simulink model "EPSArchitecture"  (R2024b)
settings: Solver=VariableStepAuto  StartTime=0.0  StopTime=10.0  RelTol=1e-3
undefined symbols (not defined in the file): I, V
settings Model: Creator=Ameya  LastModifiedBy=Ameya

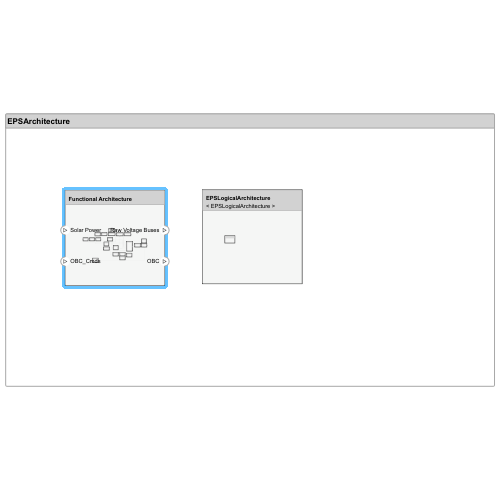
[thumbnail: Simulink's stored preview of the top-level diagram]
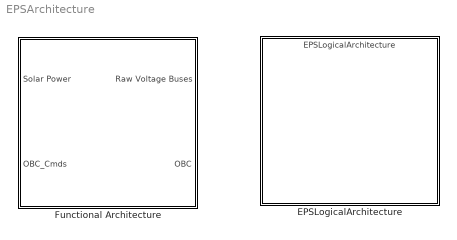
== system EPSArchitecture ==
  EPSLogicalArchitecture : ModelReference  ModelNameDialog=EPSLogicalArchitecture.slx  SimulationMode=Normal  ModelReferenceVersion=1.2
      settings: PortSchema="{\"entries\":[{\"content\":{\"headerSize\":38,\"margin\":15,\"minimumSpacing\":25,\"sides\":[{\"content\":{},\"type\":\"ConnectorPlacement.EquallySpacedRectSide\",\"uuid\":\"16a4dedc-e801-4c3c-832f-0dd2c6390a3f\"},{\"content\":{\"side\":\"RIGHT\"},\"type\":\"ConnectorPlacement.EquallySpacedRectSide\",\"uuid\":\"ee639550-12e3-4867-a673-c6f4541c780d\"},{\"content\":{\"side\":\"TOP\"},\"type\":\"ConnectorPlacement.EquallySpacedRectSide\",\"uuid\":\"10f850c7-9a2f-4ef9-b95e-dde16675c468\"}]},\"type\":\"ConnectorPlacement.EquallySpacedConnector\",\"uuid\":\"a54e4fd9-9c39-4006-b310-35c5d04543b4\"}],\"packageUris\":[\"http://schema.mathworks.com/mf0/Connector/R2020b\"],\"version\":\"1.0\"}"
  Functional Architecture : Subsystem
      settings: PortSchema="{\"entries\":[{\"content\":{\"headerSize\":26,\"margin\":15,\"minimumSpacing\":25,\"sides\":[{\"content\":{\"connectorIds\":[\"In1\",\"In2\"]},\"type\":\"ConnectorPlacement.EquallySpacedRectSide\",\"uuid\":\"94509738-6f31-4862-b12a-7ef357457276\"},{\"content\":{\"connectorIds\":[\"Out1\",\"Out2\"],\"side\":\"RIGHT\"},\"type\":\"ConnectorPlacement.EquallySpacedRectSide\",\"uuid\":\"5e6a1bf4-2d31-4a4e-ab5c-eea221f5967b\"},{\"content\":{\"side\":\"TOP\"},\"type\":\"ConnectorPlacement.EquallySpacedRectSide\",\"uuid\":\"a8cbd51e-1f9f-4875-b1c6-5db1e209e4cb\"}]},\"type\":\"ConnectorPlacement.EquallySpacedConnector\",\"uuid\":\"3c3107f4-6377-41ce-bc87-a3d6aad033f0\"}],\"packageUris\":[\"http://schema.mathworks.com/mf0/Connector/R2020b\"],\"version\":\"1.0\"}"

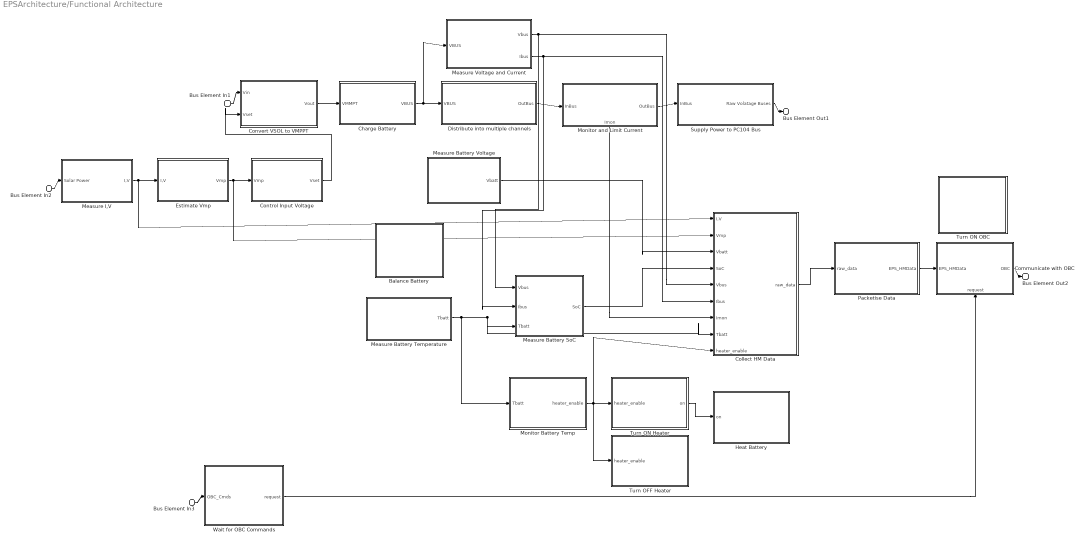
== system EPSArchitecture/Functional Architecture ==
  Bus Element In1 : Inport  PortName=Solar Power
  Bus Element In2 : Inport  PortName=Solar Power
  Bus Element In3 : Inport  Port=2  PortName=OBC_Cmds
  Balance Battery : Subsystem
      settings: PortSchema="{\"entries\":[{\"content\":{\"headerSize\":26,\"margin\":15,\"minimumSpacing\":25,\"sides\":[{\"content\":{},\"type\":\"ConnectorPlacement.EquallySpacedRectSide\",\"uuid\":\"94509738-6f31-4862-b12a-7ef357457276\"},{\"content\":{\"side\":\"RIGHT\"},\"type\":\"ConnectorPlacement.EquallySpacedRectSide\",\"uuid\":\"5e6a1bf4-2d31-4a4e-ab5c-eea221f5967b\"},{\"content\":{\"side\":\"TOP\"},\"type\":\"ConnectorPlacement.EquallySpacedRectSide\",\"uuid\":\"a8cbd51e-1f9f-4875-b1c6-5db1e209e4cb\"}]},\"type\":\"ConnectorPlacement.EquallySpacedConnector\",\"uuid\":\"3c3107f4-6377-41ce-bc87-a3d6aad033f0\"}],\"packageUris\":[\"http://schema.mathworks.com/mf0/Connector/R2020b\"],\"version\":\"1.0\"}"
  Charge Battery : Subsystem
      settings: PortSchema="{\"entries\":[{\"content\":{\"headerSize\":26,\"margin\":15,\"minimumSpacing\":25,\"sides\":[{\"content\":{\"connectorIds\":[\"In1\"]},\"type\":\"ConnectorPlacement.EquallySpacedRectSide\",\"uuid\":\"94509738-6f31-4862-b12a-7ef357457276\"},{\"content\":{\"connectorIds\":[\"Out1\"],\"side\":\"RIGHT\"},\"type\":\"ConnectorPlacement.EquallySpacedRectSide\",\"uuid\":\"5e6a1bf4-2d31-4a4e-ab5c-eea221f5967b\"},{\"content\":{\"side\":\"TOP\"},\"type\":\"ConnectorPlacement.EquallySpacedRectSide\",\"uuid\":\"a8cbd51e-1f9f-4875-b1c6-5db1e209e4cb\"}]},\"type\":\"ConnectorPlacement.EquallySpacedConnector\",\"uuid\":\"3c3107f4-6377-41ce-bc87-a3d6aad033f0\"}],\"packageUris\":[\"http://schema.mathworks.com/mf0/Connector/R2020b\"],\"version\":\"1.0\"}"
  Collect HM Data : Subsystem
      settings: PortSchema="{\"entries\":[{\"content\":{\"headerSize\":26,\"margin\":15,\"minimumSpacing\":25,\"sides\":[{\"content\":{\"connectorIds\":[\"In2\",\"In3\",\"In7\",\"In5\",\"In4\",\"In6\",\"In1\",\"In8\",\"In9\"]},\"type\":\"ConnectorPlacement.EquallySpacedRectSide\",\"uuid\":\"94509738-6f31-4862-b12a-7ef357457276\"},{\"content\":{\"connectorIds\":[\"Out1\"],\"side\":\"RIGHT\"},\"type\":\"ConnectorPlacement.EquallySpacedRectSide\",\"uuid\":\"5e6a1bf4-2d31-4a4e-ab5c-eea221f5967b\"},{\"content\":{\"side\":\"TOP\"},\"type\":\"ConnectorPlacement.EquallySpacedRectSide\",\"uuid\":\"a8cbd51e-1f9f-4875-b1c6-5db1e209e4cb\"},{\"content\":{\"side\":\"BOTTOM\"},\"type\":\"ConnectorPlacement.EquallySpacedRectSide\",\"uuid\":\"894155b8-c903-4898-a21f-10b96531ddc8\"}]},\"type\":\"ConnectorPlacement.EquallySpacedConnector\",\"uuid\":\"3c3107f4-6377-41ce-bc87-a3d6aad033f0\"}],\"packageUris\":[\"http://schema.mathworks.com/mf0/Connector/R2020b\"],\"version\":\"1.0\"}"
  Communicate with OBC : Subsystem
      settings: PortSchema="{\"entries\":[{\"content\":{\"headerSize\":26,\"margin\":15,\"minimumSpacing\":25,\"sides\":[{\"content\":{\"connectorIds\":[\"In2\"]},\"type\":\"ConnectorPlacement.EquallySpacedRectSide\",\"uuid\":\"94509738-6f31-4862-b12a-7ef357457276\"},{\"content\":{\"connectorIds\":[\"Out1\"],\"side\":\"RIGHT\"},\"type\":\"ConnectorPlacement.EquallySpacedRectSide\",\"uuid\":\"5e6a1bf4-2d31-4a4e-ab5c-eea221f5967b\"},{\"content\":{\"side\":\"TOP\"},\"type\":\"ConnectorPlacement.EquallySpacedRectSide\",\"uuid\":\"a8cbd51e-1f9f-4875-b1c6-5db1e209e4cb\"},{\"content\":{\"connectorIds\":[\"In1\"],\"side\":\"BOTTOM\"},\"type\":\"ConnectorPlacement.EquallySpacedRectSide\",\"uuid\":\"5c85cd8d-b96f-4b01-934b-f3c1b61044cb\"}]},\"type\":\"ConnectorPlacement.EquallySpacedConnector\",\"uuid\":\"3c3107f4-6377-41ce-bc87-a3d6aad033f0\"}],\"packageUris\":[\"http://schema.mathworks.com/mf0/Connector/R2020b\"],\"version\":\"1.0\"}"
  Control Input Voltage : Subsystem
      settings: PortSchema="{\"entries\":[{\"content\":{\"headerSize\":26,\"margin\":15,\"minimumSpacing\":25,\"sides\":[{\"content\":{\"connectorIds\":[\"In1\"]},\"type\":\"ConnectorPlacement.EquallySpacedRectSide\",\"uuid\":\"94509738-6f31-4862-b12a-7ef357457276\"},{\"content\":{\"connectorIds\":[\"Out1\"],\"side\":\"RIGHT\"},\"type\":\"ConnectorPlacement.EquallySpacedRectSide\",\"uuid\":\"5e6a1bf4-2d31-4a4e-ab5c-eea221f5967b\"},{\"content\":{\"side\":\"TOP\"},\"type\":\"ConnectorPlacement.EquallySpacedRectSide\",\"uuid\":\"a8cbd51e-1f9f-4875-b1c6-5db1e209e4cb\"}]},\"type\":\"ConnectorPlacement.EquallySpacedConnector\",\"uuid\":\"3c3107f4-6377-41ce-bc87-a3d6aad033f0\"}],\"packageUris\":[\"http://schema.mathworks.com/mf0/Connector/R2020b\"],\"version\":\"1.0\"}"
  Convert VSOL to VMPPT : Subsystem
      settings: PortSchema="{\"entries\":[{\"content\":{\"headerSize\":26,\"margin\":15,\"minimumSpacing\":25,\"sides\":[{\"content\":{\"connectorIds\":[\"In2\",\"In1\"]},\"type\":\"ConnectorPlacement.EquallySpacedRectSide\",\"uuid\":\"94509738-6f31-4862-b12a-7ef357457276\"},{\"content\":{\"connectorIds\":[\"Out1\"],\"side\":\"RIGHT\"},\"type\":\"ConnectorPlacement.EquallySpacedRectSide\",\"uuid\":\"5e6a1bf4-2d31-4a4e-ab5c-eea221f5967b\"},{\"content\":{\"side\":\"TOP\"},\"type\":\"ConnectorPlacement.EquallySpacedRectSide\",\"uuid\":\"a8cbd51e-1f9f-4875-b1c6-5db1e209e4cb\"},{\"content\":{\"side\":\"BOTTOM\"},\"type\":\"ConnectorPlacement.EquallySpacedRectSide\",\"uuid\":\"4bc2357f-6cbf-4a1a-8384-978abe31c3d6\"}]},\"type\":\"ConnectorPlacement.EquallySpacedConnector\",\"uuid\":\"3c3107f4-6377-41ce-bc87-a3d6aad033f0\"}],\"packageUris\":[\"http://schema.mathworks.com/mf0/Connector/R2020b\"],\"version\":\"1.0\"}"
  Distribute into multiple channels : Subsystem
      settings: PortSchema="{\"entries\":[{\"content\":{\"headerSize\":26,\"margin\":15,\"minimumSpacing\":25,\"sides\":[{\"content\":{\"connectorIds\":[\"In1\"]},\"type\":\"ConnectorPlacement.EquallySpacedRectSide\",\"uuid\":\"94509738-6f31-4862-b12a-7ef357457276\"},{\"content\":{\"connectorIds\":[\"Out1\"],\"side\":\"RIGHT\"},\"type\":\"ConnectorPlacement.EquallySpacedRectSide\",\"uuid\":\"5e6a1bf4-2d31-4a4e-ab5c-eea221f5967b\"},{\"content\":{\"side\":\"TOP\"},\"type\":\"ConnectorPlacement.EquallySpacedRectSide\",\"uuid\":\"a8cbd51e-1f9f-4875-b1c6-5db1e209e4cb\"},{\"content\":{\"side\":\"BOTTOM\"},\"type\":\"ConnectorPlacement.EquallySpacedRectSide\",\"uuid\":\"75e56ff6-a338-4e40-9de2-d2fe93eef496\"}]},\"type\":\"ConnectorPlacement.EquallySpacedConnector\",\"uuid\":\"3c3107f4-6377-41ce-bc87-a3d6aad033f0\"}],\"packageUris\":[\"http://schema.mathworks.com/mf0/Connector/R2020b\"],\"version\":\"1.0\"}"
  Estimate Vmp : Subsystem
      settings: PortSchema="{\"entries\":[{\"content\":{\"headerSize\":26,\"margin\":15,\"minimumSpacing\":25,\"sides\":[{\"content\":{\"connectorIds\":[\"In1\"]},\"type\":\"ConnectorPlacement.EquallySpacedRectSide\",\"uuid\":\"94509738-6f31-4862-b12a-7ef357457276\"},{\"content\":{\"connectorIds\":[\"Out1\"],\"side\":\"RIGHT\"},\"type\":\"ConnectorPlacement.EquallySpacedRectSide\",\"uuid\":\"5e6a1bf4-2d31-4a4e-ab5c-eea221f5967b\"},{\"content\":{\"side\":\"TOP\"},\"type\":\"ConnectorPlacement.EquallySpacedRectSide\",\"uuid\":\"a8cbd51e-1f9f-4875-b1c6-5db1e209e4cb\"}]},\"type\":\"ConnectorPlacement.EquallySpacedConnector\",\"uuid\":\"3c3107f4-6377-41ce-bc87-a3d6aad033f0\"}],\"packageUris\":[\"http://schema.mathworks.com/mf0/Connector/R2020b\"],\"version\":\"1.0\"}"
  Heat Battery : Subsystem
      settings: PortSchema="{\"entries\":[{\"content\":{\"headerSize\":26,\"margin\":15,\"minimumSpacing\":25,\"sides\":[{\"content\":{\"connectorIds\":[\"In1\"]},\"type\":\"ConnectorPlacement.EquallySpacedRectSide\",\"uuid\":\"94509738-6f31-4862-b12a-7ef357457276\"},{\"content\":{\"side\":\"RIGHT\"},\"type\":\"ConnectorPlacement.EquallySpacedRectSide\",\"uuid\":\"5e6a1bf4-2d31-4a4e-ab5c-eea221f5967b\"},{\"content\":{\"side\":\"TOP\"},\"type\":\"ConnectorPlacement.EquallySpacedRectSide\",\"uuid\":\"a8cbd51e-1f9f-4875-b1c6-5db1e209e4cb\"}]},\"type\":\"ConnectorPlacement.EquallySpacedConnector\",\"uuid\":\"3c3107f4-6377-41ce-bc87-a3d6aad033f0\"}],\"packageUris\":[\"http://schema.mathworks.com/mf0/Connector/R2020b\"],\"version\":\"1.0\"}"
  Measure Battery SoC : Subsystem
      settings: PortSchema="{\"entries\":[{\"content\":{\"headerSize\":26,\"margin\":15,\"minimumSpacing\":25,\"sides\":[{\"content\":{\"connectorIds\":[\"In1\",\"In2\",\"In3\"]},\"type\":\"ConnectorPlacement.EquallySpacedRectSide\",\"uuid\":\"94509738-6f31-4862-b12a-7ef357457276\"},{\"content\":{\"connectorIds\":[\"Out1\"],\"side\":\"RIGHT\"},\"type\":\"ConnectorPlacement.EquallySpacedRectSide\",\"uuid\":\"5e6a1bf4-2d31-4a4e-ab5c-eea221f5967b\"},{\"content\":{\"side\":\"TOP\"},\"type\":\"ConnectorPlacement.EquallySpacedRectSide\",\"uuid\":\"a8cbd51e-1f9f-4875-b1c6-5db1e209e4cb\"}]},\"type\":\"ConnectorPlacement.EquallySpacedConnector\",\"uuid\":\"3c3107f4-6377-41ce-bc87-a3d6aad033f0\"}],\"packageUris\":[\"http://schema.mathworks.com/mf0/Connector/R2020b\"],\"version\":\"1.0\"}"
  Measure Battery Temperature : Subsystem
      settings: PortSchema="{\"entries\":[{\"content\":{\"headerSize\":26,\"margin\":15,\"minimumSpacing\":25,\"sides\":[{\"content\":{},\"type\":\"ConnectorPlacement.EquallySpacedRectSide\",\"uuid\":\"94509738-6f31-4862-b12a-7ef357457276\"},{\"content\":{\"connectorIds\":[\"Out1\"],\"side\":\"RIGHT\"},\"type\":\"ConnectorPlacement.EquallySpacedRectSide\",\"uuid\":\"5e6a1bf4-2d31-4a4e-ab5c-eea221f5967b\"},{\"content\":{\"side\":\"TOP\"},\"type\":\"ConnectorPlacement.EquallySpacedRectSide\",\"uuid\":\"a8cbd51e-1f9f-4875-b1c6-5db1e209e4cb\"}]},\"type\":\"ConnectorPlacement.EquallySpacedConnector\",\"uuid\":\"3c3107f4-6377-41ce-bc87-a3d6aad033f0\"}],\"packageUris\":[\"http://schema.mathworks.com/mf0/Connector/R2020b\"],\"version\":\"1.0\"}"
  Measure Battery Voltage : Subsystem
      settings: PortSchema="{\"entries\":[{\"content\":{\"headerSize\":26,\"margin\":15,\"minimumSpacing\":25,\"sides\":[{\"content\":{},\"type\":\"ConnectorPlacement.EquallySpacedRectSide\",\"uuid\":\"94509738-6f31-4862-b12a-7ef357457276\"},{\"content\":{\"connectorIds\":[\"Out1\"],\"side\":\"RIGHT\"},\"type\":\"ConnectorPlacement.EquallySpacedRectSide\",\"uuid\":\"5e6a1bf4-2d31-4a4e-ab5c-eea221f5967b\"},{\"content\":{\"side\":\"TOP\"},\"type\":\"ConnectorPlacement.EquallySpacedRectSide\",\"uuid\":\"a8cbd51e-1f9f-4875-b1c6-5db1e209e4cb\"}]},\"type\":\"ConnectorPlacement.EquallySpacedConnector\",\"uuid\":\"3c3107f4-6377-41ce-bc87-a3d6aad033f0\"}],\"packageUris\":[\"http://schema.mathworks.com/mf0/Connector/R2020b\"],\"version\":\"1.0\"}"
  Measure I,V : Subsystem
      settings: PortSchema="{\"entries\":[{\"content\":{\"headerSize\":26,\"margin\":15,\"minimumSpacing\":25,\"sides\":[{\"content\":{\"connectorIds\":[\"In1\"]},\"type\":\"ConnectorPlacement.EquallySpacedRectSide\",\"uuid\":\"94509738-6f31-4862-b12a-7ef357457276\"},{\"content\":{\"connectorIds\":[\"Out1\"],\"side\":\"RIGHT\"},\"type\":\"ConnectorPlacement.EquallySpacedRectSide\",\"uuid\":\"5e6a1bf4-2d31-4a4e-ab5c-eea221f5967b\"},{\"content\":{\"side\":\"TOP\"},\"type\":\"ConnectorPlacement.EquallySpacedRectSide\",\"uuid\":\"a8cbd51e-1f9f-4875-b1c6-5db1e209e4cb\"},{\"content\":{\"side\":\"BOTTOM\"},\"type\":\"ConnectorPlacement.EquallySpacedRectSide\",\"uuid\":\"098d25a9-921a-42c9-a2dc-9e741d9c99a6\"}]},\"type\":\"ConnectorPlacement.EquallySpacedConnector\",\"uuid\":\"3c3107f4-6377-41ce-bc87-a3d6aad033f0\"}],\"packageUris\":[\"http://schema.mathworks.com/mf0/Connector/R2020b\"],\"version\":\"1.0\"}"
  Measure Voltage and Current : Subsystem
      settings: PortSchema="{\"entries\":[{\"content\":{\"headerSize\":26,\"margin\":15,\"minimumSpacing\":25,\"sides\":[{\"content\":{\"connectorIds\":[\"In1\"]},\"type\":\"ConnectorPlacement.EquallySpacedRectSide\",\"uuid\":\"94509738-6f31-4862-b12a-7ef357457276\"},{\"content\":{\"connectorIds\":[\"Out1\",\"Out2\"],\"side\":\"RIGHT\"},\"type\":\"ConnectorPlacement.EquallySpacedRectSide\",\"uuid\":\"5e6a1bf4-2d31-4a4e-ab5c-eea221f5967b\"},{\"content\":{\"side\":\"TOP\"},\"type\":\"ConnectorPlacement.EquallySpacedRectSide\",\"uuid\":\"a8cbd51e-1f9f-4875-b1c6-5db1e209e4cb\"}]},\"type\":\"ConnectorPlacement.EquallySpacedConnector\",\"uuid\":\"3c3107f4-6377-41ce-bc87-a3d6aad033f0\"}],\"packageUris\":[\"http://schema.mathworks.com/mf0/Connector/R2020b\"],\"version\":\"1.0\"}"
  Monitor Battery Temp : Subsystem
      settings: PortSchema="{\"entries\":[{\"content\":{\"headerSize\":26,\"margin\":15,\"minimumSpacing\":25,\"sides\":[{\"content\":{\"connectorIds\":[\"In1\"]},\"type\":\"ConnectorPlacement.EquallySpacedRectSide\",\"uuid\":\"94509738-6f31-4862-b12a-7ef357457276\"},{\"content\":{\"connectorIds\":[\"Out1\"],\"side\":\"RIGHT\"},\"type\":\"ConnectorPlacement.EquallySpacedRectSide\",\"uuid\":\"5e6a1bf4-2d31-4a4e-ab5c-eea221f5967b\"},{\"content\":{\"side\":\"TOP\"},\"type\":\"ConnectorPlacement.EquallySpacedRectSide\",\"uuid\":\"a8cbd51e-1f9f-4875-b1c6-5db1e209e4cb\"}]},\"type\":\"ConnectorPlacement.EquallySpacedConnector\",\"uuid\":\"3c3107f4-6377-41ce-bc87-a3d6aad033f0\"}],\"packageUris\":[\"http://schema.mathworks.com/mf0/Connector/R2020b\"],\"version\":\"1.0\"}"
  Monitor and Limit Current : Subsystem
      settings: PortSchema="{\"entries\":[{\"content\":{\"headerSize\":26,\"margin\":15,\"minimumSpacing\":25,\"sides\":[{\"content\":{\"connectorIds\":[\"In1\"]},\"type\":\"ConnectorPlacement.EquallySpacedRectSide\",\"uuid\":\"94509738-6f31-4862-b12a-7ef357457276\"},{\"content\":{\"connectorIds\":[\"Out2\"],\"side\":\"RIGHT\"},\"type\":\"ConnectorPlacement.EquallySpacedRectSide\",\"uuid\":\"5e6a1bf4-2d31-4a4e-ab5c-eea221f5967b\"},{\"content\":{\"side\":\"TOP\"},\"type\":\"ConnectorPlacement.EquallySpacedRectSide\",\"uuid\":\"a8cbd51e-1f9f-4875-b1c6-5db1e209e4cb\"},{\"content\":{\"connectorIds\":[\"Out1\"],\"side\":\"BOTTOM\"},\"type\":\"ConnectorPlacement.EquallySpacedRectSide\",\"uuid\":\"8debe65c-f53a-4424-8ba6-4794c80811fd\"}]},\"type\":\"ConnectorPlacement.EquallySpacedConnector\",\"uuid\":\"3c3107f4-6377-41ce-bc87-a3d6aad033f0\"}],\"packageUris\":[\"http://schema.mathworks.com/mf0/Connector/R2020b\"],\"version\":\"1.0\"}"
  Packetise Data : Subsystem
      settings: PortSchema="{\"entries\":[{\"content\":{\"headerSize\":26,\"margin\":15,\"minimumSpacing\":25,\"sides\":[{\"content\":{\"connectorIds\":[\"In1\"]},\"type\":\"ConnectorPlacement.EquallySpacedRectSide\",\"uuid\":\"94509738-6f31-4862-b12a-7ef357457276\"},{\"content\":{\"connectorIds\":[\"Out1\"],\"side\":\"RIGHT\"},\"type\":\"ConnectorPlacement.EquallySpacedRectSide\",\"uuid\":\"5e6a1bf4-2d31-4a4e-ab5c-eea221f5967b\"},{\"content\":{\"side\":\"TOP\"},\"type\":\"ConnectorPlacement.EquallySpacedRectSide\",\"uuid\":\"a8cbd51e-1f9f-4875-b1c6-5db1e209e4cb\"},{\"content\":{\"side\":\"BOTTOM\"},\"type\":\"ConnectorPlacement.EquallySpacedRectSide\",\"uuid\":\"1a7e24bf-c332-4703-81dd-0367627b027b\"}]},\"type\":\"ConnectorPlacement.EquallySpacedConnector\",\"uuid\":\"3c3107f4-6377-41ce-bc87-a3d6aad033f0\"}],\"packageUris\":[\"http://schema.mathworks.com/mf0/Connector/R2020b\"],\"version\":\"1.0\"}"
  Supply Power to PC104 Bus : Subsystem
      settings: PortSchema="{\"entries\":[{\"content\":{\"headerSize\":26,\"margin\":15,\"minimumSpacing\":25,\"sides\":[{\"content\":{\"connectorIds\":[\"In1\"]},\"type\":\"ConnectorPlacement.EquallySpacedRectSide\",\"uuid\":\"94509738-6f31-4862-b12a-7ef357457276\"},{\"content\":{\"connectorIds\":[\"Out1\"],\"side\":\"RIGHT\"},\"type\":\"ConnectorPlacement.EquallySpacedRectSide\",\"uuid\":\"5e6a1bf4-2d31-4a4e-ab5c-eea221f5967b\"},{\"content\":{\"side\":\"TOP\"},\"type\":\"ConnectorPlacement.EquallySpacedRectSide\",\"uuid\":\"a8cbd51e-1f9f-4875-b1c6-5db1e209e4cb\"}]},\"type\":\"ConnectorPlacement.EquallySpacedConnector\",\"uuid\":\"3c3107f4-6377-41ce-bc87-a3d6aad033f0\"}],\"packageUris\":[\"http://schema.mathworks.com/mf0/Connector/R2020b\"],\"version\":\"1.0\"}"
  Turn OFF Heater : Subsystem
      settings: PortSchema="{\"entries\":[{\"content\":{\"headerSize\":26,\"margin\":15,\"minimumSpacing\":25,\"sides\":[{\"content\":{\"connectorIds\":[\"In1\"]},\"type\":\"ConnectorPlacement.EquallySpacedRectSide\",\"uuid\":\"94509738-6f31-4862-b12a-7ef357457276\"},{\"content\":{\"side\":\"RIGHT\"},\"type\":\"ConnectorPlacement.EquallySpacedRectSide\",\"uuid\":\"5e6a1bf4-2d31-4a4e-ab5c-eea221f5967b\"},{\"content\":{\"side\":\"TOP\"},\"type\":\"ConnectorPlacement.EquallySpacedRectSide\",\"uuid\":\"a8cbd51e-1f9f-4875-b1c6-5db1e209e4cb\"},{\"content\":{\"side\":\"BOTTOM\"},\"type\":\"ConnectorPlacement.EquallySpacedRectSide\",\"uuid\":\"5c4ffb61-ffc3-423d-bf83-d204333b9376\"}]},\"type\":\"ConnectorPlacement.EquallySpacedConnector\",\"uuid\":\"3c3107f4-6377-41ce-bc87-a3d6aad033f0\"}],\"packageUris\":[\"http://schema.mathworks.com/mf0/Connector/R2020b\"],\"version\":\"1.0\"}"
  Turn ON Heater : Subsystem
      settings: PortSchema="{\"entries\":[{\"content\":{\"headerSize\":26,\"margin\":15,\"minimumSpacing\":25,\"sides\":[{\"content\":{\"connectorIds\":[\"In1\"]},\"type\":\"ConnectorPlacement.EquallySpacedRectSide\",\"uuid\":\"94509738-6f31-4862-b12a-7ef357457276\"},{\"content\":{\"connectorIds\":[\"Out1\"],\"side\":\"RIGHT\"},\"type\":\"ConnectorPlacement.EquallySpacedRectSide\",\"uuid\":\"5e6a1bf4-2d31-4a4e-ab5c-eea221f5967b\"},{\"content\":{\"side\":\"TOP\"},\"type\":\"ConnectorPlacement.EquallySpacedRectSide\",\"uuid\":\"a8cbd51e-1f9f-4875-b1c6-5db1e209e4cb\"}]},\"type\":\"ConnectorPlacement.EquallySpacedConnector\",\"uuid\":\"3c3107f4-6377-41ce-bc87-a3d6aad033f0\"}],\"packageUris\":[\"http://schema.mathworks.com/mf0/Connector/R2020b\"],\"version\":\"1.0\"}"
  Turn ON OBC : Subsystem
      settings: PortSchema="{\"entries\":[{\"content\":{\"headerSize\":26,\"margin\":15,\"minimumSpacing\":25,\"sides\":[{\"content\":{},\"type\":\"ConnectorPlacement.EquallySpacedRectSide\",\"uuid\":\"94509738-6f31-4862-b12a-7ef357457276\"},{\"content\":{\"side\":\"RIGHT\"},\"type\":\"ConnectorPlacement.EquallySpacedRectSide\",\"uuid\":\"5e6a1bf4-2d31-4a4e-ab5c-eea221f5967b\"},{\"content\":{\"side\":\"TOP\"},\"type\":\"ConnectorPlacement.EquallySpacedRectSide\",\"uuid\":\"a8cbd51e-1f9f-4875-b1c6-5db1e209e4cb\"}]},\"type\":\"ConnectorPlacement.EquallySpacedConnector\",\"uuid\":\"3c3107f4-6377-41ce-bc87-a3d6aad033f0\"}],\"packageUris\":[\"http://schema.mathworks.com/mf0/Connector/R2020b\"],\"version\":\"1.0\"}"
  Wait for OBC Commands : Subsystem
      settings: PortSchema="{\"entries\":[{\"content\":{\"headerSize\":26,\"margin\":15,\"minimumSpacing\":25,\"sides\":[{\"content\":{\"connectorIds\":[\"In1\"]},\"type\":\"ConnectorPlacement.EquallySpacedRectSide\",\"uuid\":\"94509738-6f31-4862-b12a-7ef357457276\"},{\"content\":{\"connectorIds\":[\"Out1\"],\"side\":\"RIGHT\"},\"type\":\"ConnectorPlacement.EquallySpacedRectSide\",\"uuid\":\"5e6a1bf4-2d31-4a4e-ab5c-eea221f5967b\"},{\"content\":{\"side\":\"TOP\"},\"type\":\"ConnectorPlacement.EquallySpacedRectSide\",\"uuid\":\"a8cbd51e-1f9f-4875-b1c6-5db1e209e4cb\"}]},\"type\":\"ConnectorPlacement.EquallySpacedConnector\",\"uuid\":\"3c3107f4-6377-41ce-bc87-a3d6aad033f0\"}],\"packageUris\":[\"http://schema.mathworks.com/mf0/Connector/R2020b\"],\"version\":\"1.0\"}"
  Bus Element Out1 : Outport  PortName=Raw Voltage Buses
  Bus Element Out2 : Outport  Port=2  PortName=OBC
  wires:
  Convert VSOL to VMPPT/1(Vout) -> Charge Battery/1(VMMPT)
  Bus Element In1/1 -> Convert VSOL to VMPPT/2(Vin)
  Bus Element In2/1 -> Measure I,V/1(Solar Power)
  Measure I,V/1(I,V) -> Collect HM Data/2(I,V), Estimate Vmp/1(I,V)
  Control Input Voltage/1(Vset) -> Convert VSOL to VMPPT/1(Vset)
  Estimate Vmp/1(Vmp) -> Collect HM Data/3(Vmp), Control Input Voltage/1(Vmp)
  Charge Battery/1(VBUS) -> Measure Voltage and Current/1(VBUS), Distribute into multiple channels/1(VBUS)
  Distribute into multiple channels/1(OutBus) -> Monitor and Limit Current/1(InBus)
  Monitor and Limit Current/2(OutBus) -> Supply Power to PC104 Bus/1(InBus)
  Supply Power to PC104 Bus/1(Raw Volatage Buses) -> Bus Element Out1/1
  Measure Battery Voltage/1(Vbatt) -> Collect HM Data/7(Vbatt)
  Monitor and Limit Current/1(Imon) -> Collect HM Data/1(Imon)
  Measure Battery SoC/1(SoC) -> Collect HM Data/5(SoC)
  Measure Voltage and Current/1(Vbus) -> Measure Battery SoC/1(Vbus), Collect HM Data/4(Vbus)
  Collect HM Data/1(raw_data) -> Packetise Data/1(raw_data)
  Packetise Data/1(EPS_HMData) -> Communicate with OBC/2(EPS_HMData)
  Communicate with OBC/1(OBC) -> Bus Element Out2/1
  Measure Voltage and Current/2(Ibus) -> Measure Battery SoC/2(Ibus), Collect HM Data/6(Ibus)
  Measure Battery Temperature/1(Tbatt) -> Monitor Battery Temp/1(Tbatt), Collect HM Data/8(Tbatt), Measure Battery SoC/3(Tbatt)
  Monitor Battery Temp/1(heater_enable) -> Collect HM Data/9(heater_enable), Turn OFF Heater/1(heater_enable), Turn ON Heater/1(heater_enable)
  Turn ON Heater/1(on) -> Heat Battery/1(on)
  Wait for OBC Commands/1(request) -> Communicate with OBC/1(request)
  Bus Element In3/1 -> Wait for OBC Commands/1(OBC_Cmds)

== system EPSArchitecture/Functional Architecture/Balance Battery ==

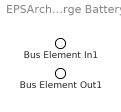
== system EPSArchitecture/Functional Architecture/Charge Battery ==
  Bus Element In1 : Inport  PortName=VMMPT
  Bus Element Out1 : Outport  PortName=VBUS

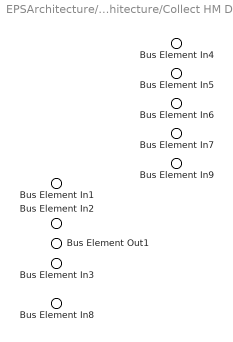
== system EPSArchitecture/Functional Architecture/Collect HM Data ==
  Bus Element In4 : Inport  PortName=Imon
  Bus Element In1 : Inport  Port=2  PortName=I,V
  Bus Element In2 : Inport  Port=3  PortName=Vmp
  Bus Element In6 : Inport  Port=4  PortName=Vbus
  Bus Element In5 : Inport  Port=5  PortName=SoC
  Bus Element In7 : Inport  Port=6  PortName=Ibus
  Bus Element In3 : Inport  Port=7  PortName=Vbatt
  Bus Element In9 : Inport  Port=8  PortName=Tbatt
  Bus Element In8 : Inport  Port=9  PortName=heater_enable
  Bus Element Out1 : Outport  PortName=raw_data

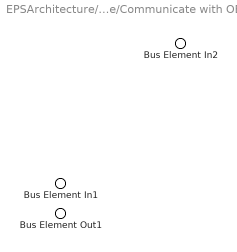
== system EPSArchitecture/Functional Architecture/Communicate with OBC ==
  Bus Element In2 : Inport  PortName=request
  Bus Element In1 : Inport  Port=2  PortName=EPS_HMData
  Bus Element Out1 : Outport  PortName=OBC

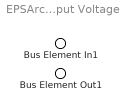
== system EPSArchitecture/Functional Architecture/Control Input Voltage ==
  Bus Element In1 : Inport  PortName=Vmp
  Bus Element Out1 : Outport  PortName=Vset

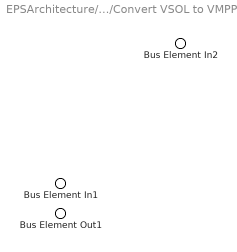
== system EPSArchitecture/Functional Architecture/Convert VSOL to VMPPT ==
  Bus Element In2 : Inport  PortName=Vset
  Bus Element In1 : Inport  Port=2  PortName=Vin
  Bus Element Out1 : Outport  PortName=Vout

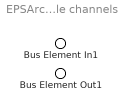
== system EPSArchitecture/Functional Architecture/Distribute into multiple channels ==
  Bus Element In1 : Inport  PortName=VBUS
  Bus Element Out1 : Outport  PortName=OutBus

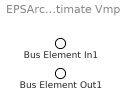
== system EPSArchitecture/Functional Architecture/Estimate Vmp ==
  Bus Element In1 : Inport  PortName=I,V
  Bus Element Out1 : Outport  PortName=Vmp

== system EPSArchitecture/Functional Architecture/Heat Battery ==
  Bus Element In1 : Inport  PortName=on

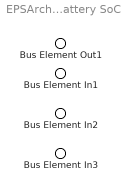
== system EPSArchitecture/Functional Architecture/Measure Battery SoC ==
  Bus Element In1 : Inport  PortName=Vbus
  Bus Element In2 : Inport  Port=2  PortName=Ibus
  Bus Element In3 : Inport  Port=3  PortName=Tbatt
  Bus Element Out1 : Outport  PortName=SoC

== system EPSArchitecture/Functional Architecture/Measure Battery Temperature ==
  Bus Element Out1 : Outport  PortName=Tbatt

== system EPSArchitecture/Functional Architecture/Measure Battery Voltage ==
  Bus Element Out1 : Outport  PortName=Vbatt

== system EPSArchitecture/Functional Architecture/Measure I,V ==
  Bus Element In1 : Inport  PortName=Solar Power
  Bus Element Out2 : Outport  PortName=I,V

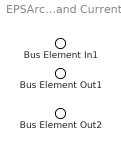
== system EPSArchitecture/Functional Architecture/Measure Voltage and Current ==
  Bus Element In1 : Inport  PortName=VBUS
  Bus Element Out1 : Outport  PortName=Vbus
  Bus Element Out2 : Outport  Port=2  PortName=Ibus

== system EPSArchitecture/Functional Architecture/Monitor Battery Temp ==
  Bus Element In1 : Inport  PortName=Tbatt
  Bus Element Out1 : Outport  PortName=heater_enable

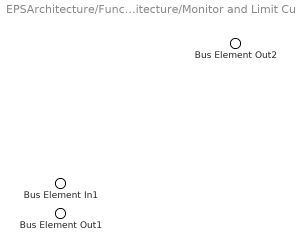
== system EPSArchitecture/Functional Architecture/Monitor and Limit Current ==
  Bus Element In1 : Inport  PortName=InBus
  Bus Element Out2 : Outport  PortName=Imon
  Bus Element Out1 : Outport  Port=2  PortName=OutBus

== system EPSArchitecture/Functional Architecture/Packetise Data ==
  Bus Element In1 : Inport  PortName=raw_data
  Bus Element Out1 : Outport  PortName=EPS_HMData

== system EPSArchitecture/Functional Architecture/Supply Power to PC104 Bus ==
  Bus Element In1 : Inport  PortName=InBus
  Bus Element Out1 : Outport  PortName=Raw Volatage Buses

== system EPSArchitecture/Functional Architecture/Turn OFF Heater ==
  Bus Element In1 : Inport  PortName=heater_enable

== system EPSArchitecture/Functional Architecture/Turn ON Heater ==
  Bus Element In1 : Inport  PortName=heater_enable
  Bus Element Out1 : Outport  PortName=on

== system EPSArchitecture/Functional Architecture/Turn ON OBC ==

== system EPSArchitecture/Functional Architecture/Wait for OBC Commands ==
  Bus Element In1 : Inport  PortName=OBC_Cmds
  Bus Element Out1 : Outport  PortName=request
